simulink model "quad_state_sensor_noise"  (R2021a)
settings: Solver=FixedStepAuto  StartTime=0.0  StopTime=sim_time  FixedStep=1/sim_freq  RelTol=1e-3
undefined symbols (not defined in the file): drift_factor, drift_tau, omega_b_bias, omega_b_noise, pos_e_noise, quat_noise, sim_freq, vel_e_bias, vel_e_noise
libraries: simulink x10, sharedutil x1
settings Model: Creator=anton  LastModifiedBy=esl
settings SolverCC: AlgebraicLoopSolver=TrustRegion
settings DebuggingCC: SFMachineParentedDataDiag=warning
settings SFSimCC: CustomCodeUndefinedFunction=UseInterfaceOnly

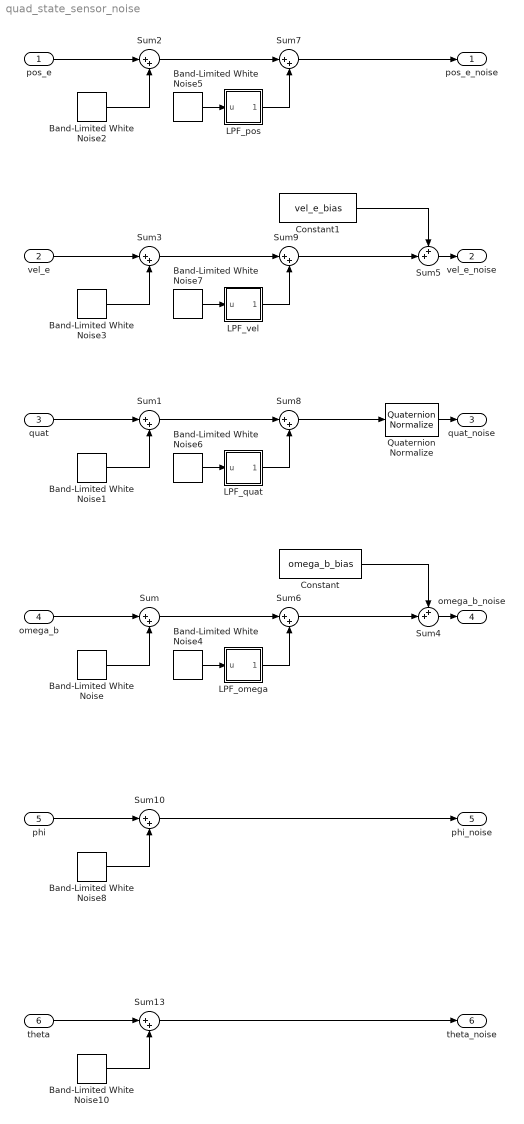
== system quad_state_sensor_noise ==
  pos_e : Inport  PortDimensions=3
  vel_e : Inport  Port=2  PortDimensions=3
  quat : Inport  Port=3  PortDimensions=4
  omega_b : Inport  Port=4  PortDimensions=3
  phi : Inport  Port=5  PortDimensions=1
  theta : Inport  Port=6  PortDimensions=1
  Band-Limited White Noise : simulink/Sources/Band-Limited White Noise  Cov=omega_b_noise  Ts=1/sim_freq  seed=[2]
  Band-Limited White Noise1 : simulink/Sources/Band-Limited White Noise  Cov=quat_noise  Ts=1/sim_freq  seed=[1]
  Band-Limited White Noise10 : simulink/Sources/Band-Limited White Noise  Cov=theta_noise  Ts=1/sim_freq  seed=[4]
  Band-Limited White Noise2 : simulink/Sources/Band-Limited White Noise  Cov=pos_e_noise  Ts=1/sim_freq  seed=[11]
  Band-Limited White Noise3 : simulink/Sources/Band-Limited White Noise  Cov=vel_e_noise  Ts=1/sim_freq  seed=[6]
  Band-Limited White Noise4 : simulink/Sources/Band-Limited White Noise  Cov=omega_b_noise*drift_factor  Ts=1/sim_freq  seed=[976]
  Band-Limited White Noise5 : simulink/Sources/Band-Limited White Noise  Cov=pos_e_noise*drift_factor  Ts=1/sim_freq  seed=[33]
  Band-Limited White Noise6 : simulink/Sources/Band-Limited White Noise  Cov=quat_noise*drift_factor  Ts=1/sim_freq  seed=[841]
  Band-Limited White Noise7 : simulink/Sources/Band-Limited White Noise  Cov=vel_e_noise*drift_factor  Ts=1/sim_freq  seed=[23234]
  Band-Limited White Noise8 : simulink/Sources/Band-Limited White Noise  Cov=phi_noise  Ts=1/sim_freq  seed=[341]
  Constant : Constant  Value=omega_b_bias
  Constant1 : Constant  Value=vel_e_bias
  LPF_omega : Subsystem
  LPF_pos : Subsystem
  LPF_quat : Subsystem
  LPF_vel : Subsystem
  Quaternion Normalize : sharedutil/Quaternion Normalize  aMode=aMode
      settings: SourceProductBaseCode=AE,PW,DR,MT,UV,VE
  Sum{,1..3,6..10,13} (10 alike) : Sum  Inputs=|++
  Sum4 : Sum  Inputs=++|
  Sum5 : Sum  Inputs=++|
  pos_e_noise : Outport  PortDimensions=3  VectorParamsAs1DForOutWhenUnconnected=off
  vel_e_noise : Outport  Port=2  PortDimensions=3  VectorParamsAs1DForOutWhenUnconnected=off
  quat_noise : Outport  Port=3  PortDimensions=4  VectorParamsAs1DForOutWhenUnconnected=off
  omega_b_noise : Outport  Port=4  PortDimensions=3  VectorParamsAs1DForOutWhenUnconnected=off
  phi_noise : Outport  Port=5  VectorParamsAs1DForOutWhenUnconnected=off
  theta_noise : Outport  Port=6  VectorParamsAs1DForOutWhenUnconnected=off
  wires:
  Sum7/1 -> pos_e_noise/1
  Band-Limited White Noise2/1 -> Sum2/2
  pos_e/1 -> Sum2/1
  LPF_pos/1(u_filt) -> Sum7/2
  Sum2/1 -> Sum7/1
  Band-Limited White Noise5/1 -> LPF_pos/1(u)
  Sum5/1 -> vel_e_noise/1
  Sum9/1 -> Sum5/2
  Band-Limited White Noise3/1 -> Sum3/2
  Sum3/1 -> Sum9/1
  LPF_vel/1(u_filt) -> Sum9/2
  Constant1/1 -> Sum5/1
  vel_e/1 -> Sum3/1
  Band-Limited White Noise7/1 -> LPF_vel/1(u)
  LPF_quat/1(u_filt) -> Sum8/2
  Sum1/1 -> Sum8/1
  Sum8/1 -> Quaternion Normalize/1
  Quaternion Normalize/1 -> quat_noise/1
  Band-Limited White Noise1/1 -> Sum1/2
  quat/1 -> Sum1/1
  Band-Limited White Noise6/1 -> LPF_quat/1(u)
  Band-Limited White Noise4/1 -> LPF_omega/1(u)
  Sum/1 -> Sum6/1
  LPF_omega/1(u_filt) -> Sum6/2
  omega_b/1 -> Sum/1
  Constant/1 -> Sum4/1
  Sum4/1 -> omega_b_noise/1
  Sum6/1 -> Sum4/2
  Band-Limited White Noise/1 -> Sum/2
  Band-Limited White Noise8/1 -> Sum10/2
  Sum10/1 -> phi_noise/1
  Band-Limited White Noise10/1 -> Sum13/2
  Sum13/1 -> theta_noise/1
  theta/1 -> Sum13/1
  phi/1 -> Sum10/1

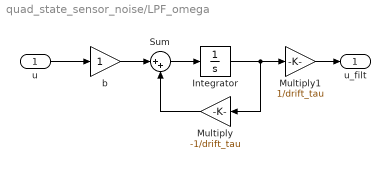
== system quad_state_sensor_noise/LPF_omega ==
  u : Inport
  Integrator : Integrator
  Multiply : Gain  Gain=-1/drift_tau
  Multiply1 : Gain  Gain=1/drift_tau
  Sum : Sum  Inputs=|++
  b : Gain
  u_filt : Outport  VectorParamsAs1DForOutWhenUnconnected=off
  wires:
  u/1 -> b/1
  b/1 -> Sum/1
  Sum/1 -> Integrator/1
  Integrator/1 -> Multiply1/1, Multiply/1
  Multiply/1 -> Sum/2
  Multiply1/1 -> u_filt/1

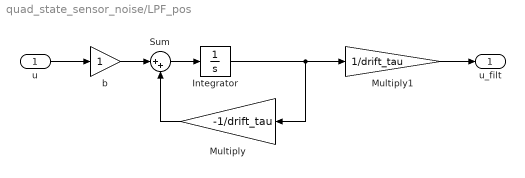
== system quad_state_sensor_noise/LPF_pos ==
  u : Inport
  Integrator : Integrator
  Multiply : Gain  Gain=-1/drift_tau
  Multiply1 : Gain  Gain=1/drift_tau
  Sum : Sum  Inputs=|++
  b : Gain
  u_filt : Outport  VectorParamsAs1DForOutWhenUnconnected=off
  wires:
  u/1 -> b/1
  b/1 -> Sum/1
  Sum/1 -> Integrator/1
  Integrator/1 -> Multiply1/1, Multiply/1
  Multiply/1 -> Sum/2
  Multiply1/1 -> u_filt/1

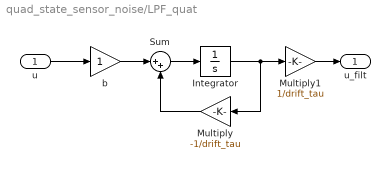
== system quad_state_sensor_noise/LPF_quat ==
  u : Inport
  Integrator : Integrator
  Multiply : Gain  Gain=-1/drift_tau
  Multiply1 : Gain  Gain=1/drift_tau
  Sum : Sum  Inputs=|++
  b : Gain
  u_filt : Outport  VectorParamsAs1DForOutWhenUnconnected=off
  wires:
  u/1 -> b/1
  b/1 -> Sum/1
  Sum/1 -> Integrator/1
  Integrator/1 -> Multiply1/1, Multiply/1
  Multiply/1 -> Sum/2
  Multiply1/1 -> u_filt/1

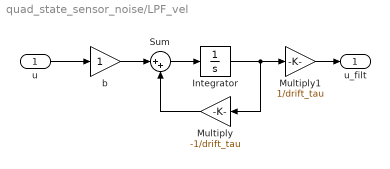
== system quad_state_sensor_noise/LPF_vel ==
  u : Inport
  Integrator : Integrator
  Multiply : Gain  Gain=-1/drift_tau
  Multiply1 : Gain  Gain=1/drift_tau
  Sum : Sum  Inputs=|++
  b : Gain
  u_filt : Outport  VectorParamsAs1DForOutWhenUnconnected=off
  wires:
  u/1 -> b/1
  b/1 -> Sum/1
  Sum/1 -> Integrator/1
  Integrator/1 -> Multiply1/1, Multiply/1
  Multiply/1 -> Sum/2
  Multiply1/1 -> u_filt/1
